simulink model "ca_interp"  (R2023b)
settings: Solver=VariableStepDiscrete  StartTime=0.0  StopTime=DUC_LINEUP_param.endTime  RelTol=1e-3  EnableMultiTasking=on
PreLoadFcn:
  | % Run the setup script when the model is opened
  | setup_ca_interp;
InitFcn:
  | % Run the setup script again just before the
  | % model is run, so that any updates made
  | % after opening are applied.
  | 
  | setup_ca_interp;
StopFcn:
  | ca_interp_output_analysis;
values from neighbouring files (symbols this model uses):
  DUC_SUMMER_multiplication_factor = 1    [setup_ca_interp.m]
  DUC_SUMMER_Number_of_bits_to_shift_left = 0    [setup_ca_interp.m]
undefined symbols (not defined in the file or in its folder): AdvDSPBChannelOutDisplay, AdvDSPBDMemDisplay, dpoly, dspba_ChannelInVis, dspba_ChannelOutVis, dspba_internal_get_channel_ports, DUC_LINEUP_param, evalAionMaskParam, latency, primtype, UseDontCare, value
libraries: DSPBAPrim x53, simulink x18, DSPBAModelBus x14, DSPBABase x12, DSPBAFilters x2
(part 2 of 2)

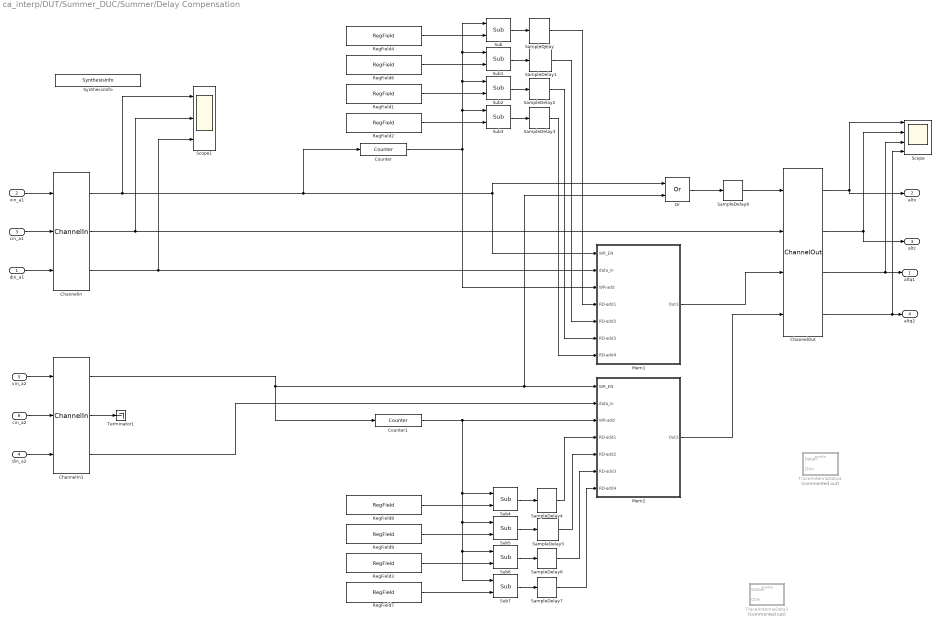
== system ca_interp/DUT/Summer_DUC/Summer/Delay Compensation ==
  din_a1 : Inport
  vin_a1 : Inport  Port=2
  cin_a1 : Inport  Port=3
  din_a2 : Inport  Port=4
  vin_a2 : Inport  Port=5
  cin_a2 : Inport  Port=6
  ChannelIn : DSPBAPrim/ChannelIn  primtype=channelin  nInputs=dspba_internal_get_channel_ports(gcb)  nOutputs=dspba_internal_get_channel_ports(gcb)  omode=Inherit via internal rule  otype=sfix(16)  scale=2^-15  rndmethod=Unbiased  factor=1  satmethod=Symmetric  shift_vec=[0 1 2 -1]  value=1  inPortNames=['v'; 'c'; '0'; '1'; '2'; '3'; '4'; '5'; '6'; '7'; '8'; '9'; 'A'; 'B'; 'D'; 'E'; 'F'; 'G'; 'H'; 'I'; 'J'; 'K'; 'L'; 'M'; 'N'; 'O'; 'P'; 'Q'; 'R'; 'S'; 'T'; 'U'; 'W'; 'X'; 'Y'; 'Z']  outPortNames=['v'; 'c'; '0'; '1'; '2'; '3'; '4'; '5'; '6'; '7'; '8'; '9'; 'A'; 'B'; 'D'; 'E'; 'F'; 'G'; 'H'; 'I'; 'J'; 'K'; 'L'; 'M'; 'N'; 'O'; 'P'; 'Q'; 'R'; 'S'; 'T'; 'U'; 'W'; 'X'; 'Y'; 'Z']  dspbaimage=dspba_prim_channel_tall.svg  text=fprintf('In');  style=Optimised  dataSignals=1  foldingEnabled=off  channels=1  sampleRate=200  packetBeginPresent=off  packetBeginEnabled=off  visibilities=dspba_ChannelInVis(gcb)  scheduleOrigin=on  version=20211214
  ChannelIn1 : DSPBAPrim/ChannelIn  primtype=channelin  nInputs=dspba_internal_get_channel_ports(gcb)  nOutputs=dspba_internal_get_channel_ports(gcb)  omode=Inherit via internal rule  otype=sfix(16)  scale=2^-15  rndmethod=Unbiased  factor=1  satmethod=Symmetric  shift_vec=[0 1 2 -1]  value=1  inPortNames=['v'; 'c'; '0'; '1'; '2'; '3'; '4'; '5'; '6'; '7'; '8'; '9'; 'A'; 'B'; 'D'; 'E'; 'F'; 'G'; 'H'; 'I'; 'J'; 'K'; 'L'; 'M'; 'N'; 'O'; 'P'; 'Q'; 'R'; 'S'; 'T'; 'U'; 'W'; 'X'; 'Y'; 'Z']  outPortNames=['v'; 'c'; '0'; '1'; '2'; '3'; '4'; '5'; '6'; '7'; '8'; '9'; 'A'; 'B'; 'D'; 'E'; 'F'; 'G'; 'H'; 'I'; 'J'; 'K'; 'L'; 'M'; 'N'; 'O'; 'P'; 'Q'; 'R'; 'S'; 'T'; 'U'; 'W'; 'X'; 'Y'; 'Z']  dspbaimage=dspba_prim_channel_tall.svg  text=fprintf('In');  style=Optimised  dataSignals=1  foldingEnabled=off  channels=1  sampleRate=200  packetBeginPresent=off  packetBeginEnabled=off  visibilities=dspba_ChannelInVis(gcb)  scheduleOrigin=on  version=20211214
  ChannelOut : DSPBAPrim/ChannelOut  primtype=channelout  nInputs=dspba_internal_get_channel_ports(gcb)  nOutputs=dspba_internal_get_channel_ports(gcb)  omode=Inherit via internal rule  otype=sfix(16)  scale=2^-15  rndmethod=Unbiased  factor=1  satmethod=Symmetric  shift_vec=[0 1 2 -1]  value=2  inPortNames=['v'; 'c'; '0'; '1'; '2'; '3'; '4'; '5'; '6'; '7'; '8'; '9'; 'A'; 'B'; 'D'; 'E'; 'F'; 'G'; 'H'; 'I'; 'J'; 'K'; 'L'; 'M'; 'N'; 'O'; 'P'; 'Q'; 'R'; 'S'; 'T'; 'U'; 'W'; 'X'; 'Y'; 'Z']  outPortNames=['v'; 'c'; '0'; '1'; '2'; '3'; '4'; '5'; '6'; '7'; '8'; '9'; 'A'; 'B'; 'D'; 'E'; 'F'; 'G'; 'H'; 'I'; 'J'; 'K'; 'L'; 'M'; 'N'; 'O'; 'P'; 'Q'; 'R'; 'S'; 'T'; 'U'; 'W'; 'X'; 'Y'; 'Z']  dspbaimage=dspba_prim_channel_tall.svg  text=fprintf('Out%s', AdvDSPBChannelOutDisplay(latency));  style=Optimised  dataSignals=2  foldingEnabled=off  channels=1  sampleRate=200  packetBeginPresent=off  packetBeginEnabled=off  visibilities=dspba_ChannelOutVis(gcb)  latency=4  version=20211214
  Counter : DSPBAPrim/Counter  primtype=counter  nInputs=1  nOutputs=1  omode=Inherit via internal rule  otype=ufix(16)  scale=2^-0  rndmethod=Unbiased  factor=1  satmethod=Symmetric  shift_vec=[0 1 2 -1]  value=[255 256 1]  inPortNames=[' '; ' ';]  outPortNames=[' ']  dspbaimage=dspba_prim.svg  text=fprintf('counter\n[%d %d %d]', value(1), value(2), value(3));  style=Optimised  visibilities=8 + 1024  version=20211007
  Counter1 : DSPBAPrim/Counter  primtype=counter  nInputs=1  nOutputs=1  omode=Inherit via internal rule  otype=ufix(16)  scale=2^-0  rndmethod=Unbiased  factor=1  satmethod=Symmetric  shift_vec=[0 1 2 -1]  value=[255 256 1]  inPortNames=[' '; ' ';]  outPortNames=[' ']  dspbaimage=dspba_prim.svg  text=fprintf('counter\n[%d %d %d]', value(1), value(2), value(3));  style=Optimised  visibilities=8 + 1024  version=20211007
  Mem1 : Subsystem
  Mem2 : Subsystem
  Or : DSPBAPrim/Or  primtype=or  nInputs=2  nOutputs=1  omode=Inherit via internal rule  otype=sfix(16)  scale=2^-15  rndmethod=Unbiased  factor=1  satmethod=Symmetric  shift_vec=[0 1 2 -1]  value=0  inPortNames=[' '; ' '; ' '; ' '; ' '; ' '; ' '; ' '; ' '; ' '; ' '; ' '; ' '; ' '; ' '; ' '; ]  outPortNames=[' ']  dspbaimage=dspba_prim.svg  text=fprintf('|');  style=Optimised  visibilities=8+2  version=20211007
  RegField1 : DSPBAModelBus/RegField  reg_name=DUC_Delay_Comp_offset_ant3_1  reg_rwmode=Read/Write  reg_msb=7  reg_lsb=0  reg_mode=Specify via dialog  reg_type=ufix(8)  reg_scale=2^0  reg_init=DUC_Delay_Comp_Ant3_CC1  reg_desc=Delay Compensation Value  reg_modal=off  reg_desc0=0  reg_desc1=0  reg_desc2=0  reg_desc3=0  reg_desc4=0  reg_desc5=0  reg_desc6=0  reg_desc7=0  reg_addr=7  SampleTime=-1  version=20090407
  RegField2 : DSPBAModelBus/RegField  reg_name=DUC_Delay_Comp_offset_ant4_1  reg_rwmode=Read/Write  reg_msb=7  reg_lsb=0  reg_mode=Specify via dialog  reg_type=ufix(8)  reg_scale=2^0  reg_init=DUC_Delay_Comp_Ant4_CC1  reg_desc=Delay Compensation Value  reg_modal=off  reg_desc0=0  reg_desc1=0  reg_desc2=0  reg_desc3=0  reg_desc4=0  reg_desc5=0  reg_desc6=0  reg_desc7=0  reg_addr=8  SampleTime=-1  version=20090407
  RegField3 : DSPBAModelBus/RegField  reg_name=DUC_Delay_Comp_offset_ant3_2  reg_rwmode=Read/Write  reg_msb=7  reg_lsb=0  reg_mode=Specify via dialog  reg_type=ufix(8)  reg_scale=2^0  reg_init=DUC_Delay_Comp_Ant3_CC2  reg_desc=Delay Compensation Value  reg_modal=off  reg_desc0=0  reg_desc1=0  reg_desc2=0  reg_desc3=0  reg_desc4=0  reg_desc5=0  reg_desc6=0  reg_desc7=0  reg_addr=11  SampleTime=-1  version=20090407
  RegField4 : DSPBAModelBus/RegField  reg_name=DUC_Delay_Comp_offset_ant1_1  reg_rwmode=Read/Write  reg_msb=7  reg_lsb=0  reg_mode=Specify via dialog  reg_type=ufix(8)  reg_scale=2^0  reg_init=DUC_Delay_Comp_Ant1_CC1  reg_desc=Delay Compensation Value  reg_modal=off  reg_desc0=0  reg_desc1=0  reg_desc2=0  reg_desc3=0  reg_desc4=0  reg_desc5=0  reg_desc6=0  reg_desc7=0  reg_addr=5  SampleTime=-1  version=20090407
  RegField6 : DSPBAModelBus/RegField  reg_name=DUC_Delay_Comp_offset_ant2_1  reg_rwmode=Read/Write  reg_msb=7  reg_lsb=0  reg_mode=Specify via dialog  reg_type=ufix(8)  reg_scale=2^0  reg_init=DUC_Delay_Comp_Ant2_CC1  reg_desc=Delay Compensation Value  reg_modal=off  reg_desc0=0  reg_desc1=0  reg_desc2=0  reg_desc3=0  reg_desc4=0  reg_desc5=0  reg_desc6=0  reg_desc7=0  reg_addr=6  SampleTime=-1  version=20090407
  RegField7 : DSPBAModelBus/RegField  reg_name=DUC_Delay_Comp_offset_ant4_2  reg_rwmode=Read/Write  reg_msb=7  reg_lsb=0  reg_mode=Specify via dialog  reg_type=ufix(8)  reg_scale=2^0  reg_init=DUC_Delay_Comp_Ant4_CC2  reg_desc=Delay Compensation Value  reg_modal=off  reg_desc0=0  reg_desc1=0  reg_desc2=0  reg_desc3=0  reg_desc4=0  reg_desc5=0  reg_desc6=0  reg_desc7=0  reg_addr=12  SampleTime=-1  version=20090407
  RegField8 : DSPBAModelBus/RegField  reg_name=DUC_Delay_Comp_offset_ant1_2  reg_rwmode=Read/Write  reg_msb=7  reg_lsb=0  reg_mode=Specify via dialog  reg_type=ufix(8)  reg_scale=2^0  reg_init=DUC_Delay_Comp_Ant1_CC2  reg_desc=Delay Compensation Value  reg_modal=off  reg_desc0=0  reg_desc1=0  reg_desc2=0  reg_desc3=0  reg_desc4=0  reg_desc5=0  reg_desc6=0  reg_desc7=0  reg_addr=9  SampleTime=-1  version=20090407
  RegField9 : DSPBAModelBus/RegField  reg_name=DUC_Delay_Comp_offset_ant2_2  reg_rwmode=Read/Write  reg_msb=7  reg_lsb=0  reg_mode=Specify via dialog  reg_type=ufix(8)  reg_scale=2^0  reg_init=DUC_Delay_Comp_Ant2_CC2  reg_desc=Delay Compensation Value  reg_modal=off  reg_desc0=0  reg_desc1=0  reg_desc2=0  reg_desc3=0  reg_desc4=0  reg_desc5=0  reg_desc6=0  reg_desc7=0  reg_addr=10  SampleTime=-1  version=20090407
  SampleDelay{,1..8} (9 alike) : DSPBAPrim/SampleDelay  primtype=sampdelay  nInputs=1  nOutputs=1  omode=Inherit via internal rule  otype=sfix(16)  scale=2^-15  rndmethod=Unbiased  factor=1  satmethod=Symmetric  shift_vec=[0 1 2 -1]  floatPrecision=float32_m23  value=2  inPortNames=[' '; ' ';]  outPortNames=[' ']  dspbaimage=dspba_prim.svg  text=dpoly(1, eye(1,value+1), 'z')  style=Optimised  visibilities=8 + 1024 + 2^17 + 2^18  flexible=off  slackgroup=0  augmented=0  version=20211007  advOptions=[]
  Scope : Scope  NumInputPorts=4
  Scope1 : Scope  NumInputPorts=3
  Sub{,1..7} (8 alike) : DSPBAPrim/Sub  primtype=sub  nInputs=2  nOutputs=1  omode=Specify via dialog  otype=uint(8)  scale=2^0  rndmethod=Unbiased  factor=1  satmethod=Symmetric  shift_vec=[0 1 2 -1]  value=0  inPortNames=['+'; '-';]  outPortNames=[' ']  dspbaimage=dspba_prim.svg  text=fprintf('-');  style=Optimised  visibilities=8+2^17+2^18  floatRounding=correct  advOptions=[]  version=20211007
  SynthesisInfo : DSPBAPrim/SynthesisInfo  primtype=synthinfo  nInputs=0  nOutputs=0  omode=Inherit via internal rule  otype=sfix(16)  scale=2^-15  rndmethod=Truncate  factor=1  satmethod=Symmetric  shift_vec=[0 1 2 -1]  value=99  inPortNames=[' '; ' ';]  outPortNames=[' ']  dspbaimage=dspba_prim_ctrl.jpg  text=fprintf('Style=%s', style);  style=Scheduled  visibilities=2^17+2^18+2^19+2^20+2^21+2^22+2^23+2^24  constraintPair=None  constraintRelation=>  constraintLimit=Latency  modelRefSign=+  modelRef=''  showSchedule=off  simulationMode=Use Global Value  resetMinimization=Conditional - On for ChannelIn/Out only  version=20220106
  Terminator1 : Terminator
  TraceAntennaData1 : Subsystem  Commented=on  TreatAsAtomicUnit=on
  TraceAntennaData4 : Subsystem  Commented=on  TreatAsAtomicUnit=on
  altq1 : Outport
  altv : Outport  Port=2
  altc : Outport  Port=3
  altq2 : Outport  Port=4
  wires:
  ChannelIn/2 -> Scope1/2, ChannelOut/2
  Counter/1 -> Mem1/3(WR-add), Sub2/1, Sub1/1, Sub/1, Sub3/1
  RegField4/1 -> Sub/2
  ChannelIn1/1 -> Counter1/1, Or/2, Mem2/1(WR_EN)
  din_a2/1 -> ChannelIn1/3
  vin_a2/1 -> ChannelIn1/1
  ChannelIn1/2 -> Terminator1/1
  cin_a2/1 -> ChannelIn1/2
  ChannelOut/3 -> Scope/3, altq1/1
  ChannelOut/2 -> Scope/2, altc/1
  ChannelOut/1 -> Scope/1, altv/1
  din_a1/1 -> ChannelIn/3
  vin_a1/1 -> ChannelIn/1
  cin_a1/1 -> ChannelIn/2
  RegField6/1 -> Sub1/2
  RegField1/1 -> Sub2/2
  RegField2/1 -> Sub3/2
  Mem1/1(Out3) -> ChannelOut/3
  Sub/1 -> SampleDelay/1
  Sub1/1 -> SampleDelay1/1
  Sub2/1 -> SampleDelay2/1
  Sub3/1 -> SampleDelay3/1
  ChannelIn/3 -> Scope1/3, Mem1/2(data_in)
  ChannelOut/4 -> Scope/4, altq2/1
  Mem2/1(Out3) -> ChannelOut/4
  ChannelIn1/3 -> Mem2/2(data_in)
  RegField8/1 -> Sub4/2
  RegField9/1 -> Sub5/2
  RegField3/1 -> Sub6/2
  RegField7/1 -> Sub7/2
  Sub4/1 -> SampleDelay4/1
  Sub5/1 -> SampleDelay5/1
  Sub6/1 -> SampleDelay6/1
  Sub7/1 -> SampleDelay7/1
  ChannelIn/1 -> Scope1/1, Or/1, Mem1/1(WR_EN), Counter/1
  SampleDelay/1 -> Mem1/4(RD-add1)
  SampleDelay1/1 -> Mem1/5(RD-add2)
  SampleDelay2/1 -> Mem1/6(RD-add3)
  SampleDelay3/1 -> Mem1/7(RD-add4)
  SampleDelay4/1 -> Mem2/4(RD-add1)
  SampleDelay6/1 -> Mem2/6(RD-add3)
  SampleDelay5/1 -> Mem2/5(RD-add2)
  SampleDelay7/1 -> Mem2/7(RD-add4)
  Counter1/1 -> Sub7/1, Sub6/1, Sub5/1, Sub4/1, Mem2/3(WR-add)
  SampleDelay8/1 -> ChannelOut/1
  Or/1 -> SampleDelay8/1

== system ca_interp/DUT/Summer_DUC/Summer/Carrier Aggregation and Gain/TraceAntennaData1 ==
  DataIn : Inport
  ChIn : Inport  Port=2
  Enable : EnablePort
  DucAntDataOut : ToWorkspace  VariableName=AntGain_dOut  SampleTime=-1
  DucAntDataOut1 : ToWorkspace  VariableName=AntGain_cOut  SampleTime=-1
  wires:
  DataIn/1 -> DucAntDataOut/1
  ChIn/1 -> DucAntDataOut1/1

== system ca_interp/DUT/Summer_DUC/Summer/Carrier Aggregation and Gain/TraceAntennaData4 ==
  DataIn : Inport
  ChIn : Inport  Port=2
  Enable : EnablePort
  DucAntDataOut : ToWorkspace  VariableName=AntGain_dIn  SampleTime=-1
  DucAntDataOut1 : ToWorkspace  VariableName=AntGain_cIn  SampleTime=-1
  wires:
  ChIn/1 -> DucAntDataOut1/1
  DataIn/1 -> DucAntDataOut/1

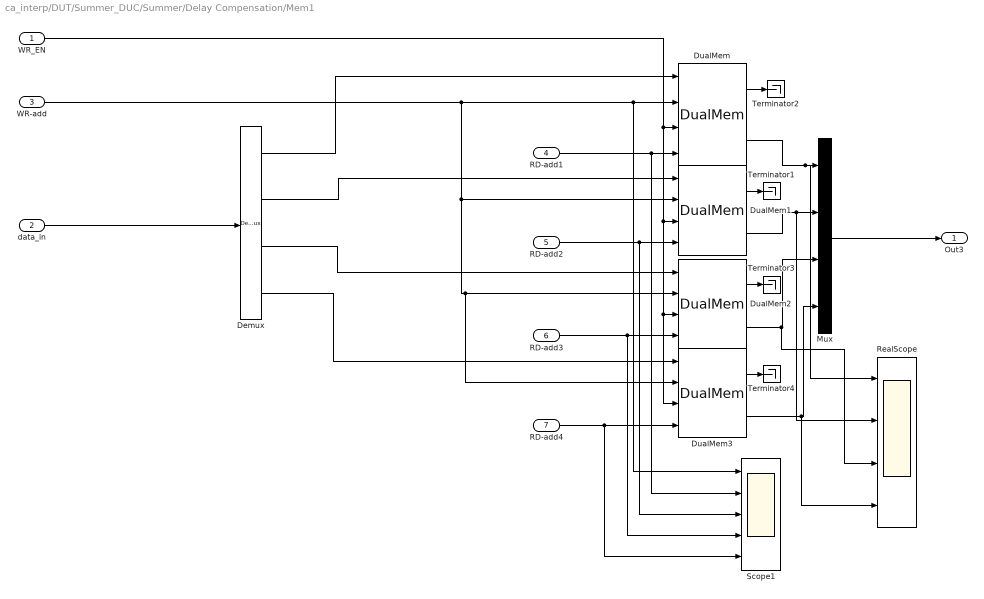
== system ca_interp/DUT/Summer_DUC/Summer/Delay Compensation/Mem1 ==
  WR_EN : Inport
  data_in : Inport  Port=2
  WR-add : Inport  Port=3
  RD-add1 : Inport  Port=4
  RD-add2 : Inport  Port=5
  RD-add3 : Inport  Port=6
  RD-add4 : Inport  Port=7
  Demux : Demux
  DualMem{,1..3} (4 alike) : DSPBAPrim/DualMem  primtype=dualmem  nInputs=4  nOutputs=2  omode=Inherit via internal rule  otype=sfix(16)  scale=2^-15  rndmethod=Unbiased  factor=1  satmethod=Symmetric  shift_vec=[0 1 2 -1]  value=[zeros(256, 1)]  inPortNames=['d1'; 'a1'; 'w1'; 'd2'; 'a2'; 'w2']  outPortNames=['q1'; 'q2']  dspbaimage=dspba_prim_tall.svg  text=fprintf('dmem%s',AdvDSPBDMemDisplay(UseDontCare));  style=Optimised  visibilities=8 + 1024 + 2^17 + 2^18  UseDontCare=on  TwinWritePorts=off  init=on  ProvideReadAccess=off  version=20211007
  Mux : Mux
  RealScope : Scope  NumInputPorts=4
  Scope1 : Scope  NumInputPorts=5
  Terminator{1..4} (4 alike) : Terminator
  Out3 : Outport
  wires:
  WR-add/1 -> Scope1/1, DualMem/2, DualMem1/2, DualMem2/2, DualMem3/2
  DualMem1/2 -> RealScope/2, Mux/2
  DualMem3/1 -> Terminator4/1
  RD-add2/1 -> Scope1/3, DualMem1/4
  DualMem2/2 -> RealScope/3, Mux/3
  Demux/4 -> DualMem3/1
  DualMem/1 -> Terminator2/1
  Demux/3 -> DualMem2/1
  RD-add3/1 -> Scope1/4, DualMem2/4
  DualMem/2 -> RealScope/1, Mux/1
  DualMem3/2 -> RealScope/4, Mux/4
  Demux/2 -> DualMem1/1
  Demux/1 -> DualMem/1
  RD-add4/1 -> Scope1/5, DualMem3/4
  Mux/1 -> Out3/1
  data_in/1 -> Demux/1
  DualMem2/1 -> Terminator3/1
  DualMem1/1 -> Terminator1/1
  WR_EN/1 -> DualMem2/3, DualMem3/3, DualMem1/3, DualMem/3
  RD-add1/1 -> Scope1/2, DualMem/4

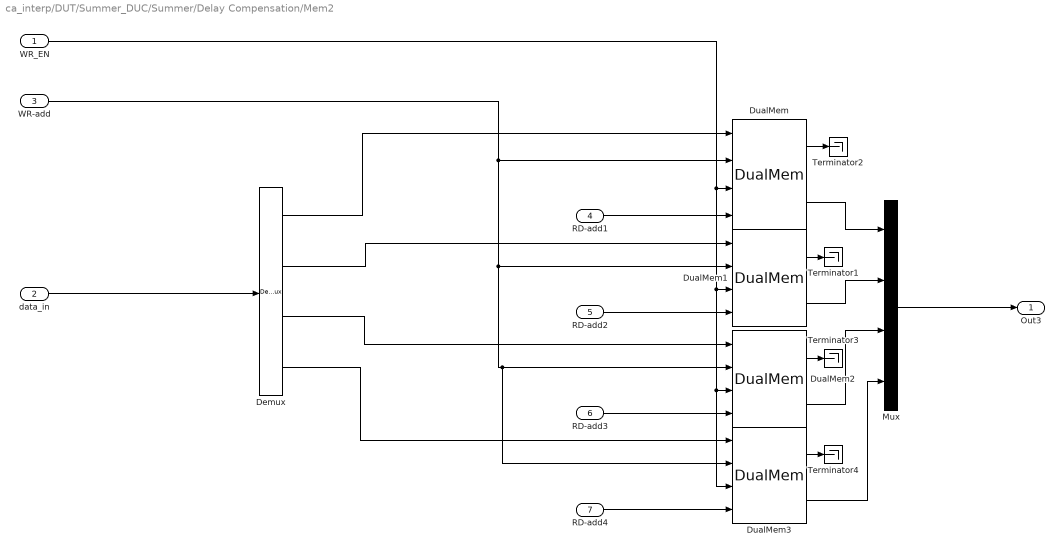
== system ca_interp/DUT/Summer_DUC/Summer/Delay Compensation/Mem2 ==
  WR_EN : Inport
  data_in : Inport  Port=2
  WR-add : Inport  Port=3
  RD-add1 : Inport  Port=4
  RD-add2 : Inport  Port=5
  RD-add3 : Inport  Port=6
  RD-add4 : Inport  Port=7
  Demux : Demux
  DualMem{,1..3} (4 alike) : DSPBAPrim/DualMem  primtype=dualmem  nInputs=4  nOutputs=2  omode=Inherit via internal rule  otype=sfix(16)  scale=2^-15  rndmethod=Unbiased  factor=1  satmethod=Symmetric  shift_vec=[0 1 2 -1]  value=[zeros(256, 1)]  inPortNames=['d1'; 'a1'; 'w1'; 'd2'; 'a2'; 'w2']  outPortNames=['q1'; 'q2']  dspbaimage=dspba_prim_tall.svg  text=fprintf('dmem%s',AdvDSPBDMemDisplay(UseDontCare));  style=Optimised  visibilities=8 + 1024 + 2^17 + 2^18  UseDontCare=on  TwinWritePorts=off  init=on  ProvideReadAccess=off  version=20211007
  Mux : Mux
  Terminator{1..4} (4 alike) : Terminator
  Out3 : Outport
  wires:
  DualMem1/1 -> Terminator1/1
  DualMem2/1 -> Terminator3/1
  data_in/1 -> Demux/1
  RD-add1/1 -> DualMem/4
  Mux/1 -> Out3/1
  RD-add4/1 -> DualMem3/4
  Demux/1 -> DualMem/1
  Demux/2 -> DualMem1/1
  DualMem3/2 -> Mux/4
  DualMem/2 -> Mux/1
  RD-add3/1 -> DualMem2/4
  Demux/3 -> DualMem2/1
  DualMem/1 -> Terminator2/1
  Demux/4 -> DualMem3/1
  DualMem2/2 -> Mux/3
  RD-add2/1 -> DualMem1/4
  DualMem3/1 -> Terminator4/1
  WR_EN/1 -> DualMem/3, DualMem1/3, DualMem3/3, DualMem2/3
  DualMem1/2 -> Mux/2
  WR-add/1 -> DualMem3/2, DualMem2/2, DualMem1/2, DualMem/2

== system ca_interp/DUT/Summer_DUC/Summer/Delay Compensation/TraceAntennaData1 ==
  DataIn : Inport
  ChIn : Inport  Port=2
  Enable : EnablePort
  DucAntDataOut : ToWorkspace  VariableName=AntGain_dOut  SampleTime=-1
  DucAntDataOut1 : ToWorkspace  VariableName=AntGain_cOut  SampleTime=-1
  wires:
  ChIn/1 -> DucAntDataOut1/1
  DataIn/1 -> DucAntDataOut/1

== system ca_interp/DUT/Summer_DUC/Summer/Delay Compensation/TraceAntennaData4 ==
  DataIn : Inport
  ChIn : Inport  Port=2
  Enable : EnablePort
  DucAntDataOut : ToWorkspace  VariableName=AntGain_dIn  SampleTime=-1
  DucAntDataOut1 : ToWorkspace  VariableName=AntGain_cIn  SampleTime=-1
  wires:
  DataIn/1 -> DucAntDataOut/1
  ChIn/1 -> DucAntDataOut1/1
